simulink model "npc_controller"  (R2022a)
settings: Solver=FixedStepDiscrete  StartTime=0.0  StopTime=20  RelTol=1e-3  EnableMultiTasking=on
undefined symbols (not defined in the file): CAN_O_INT, CANA_BASE, Down, GPTRIP1SEL, GPTRIP2SEL, GPTRIP3SEL, Tsw, TZ1, TZ2, TZ3, Up
libraries: simulink x147, hdlsllib x90, c2802xlib x34, c2837xDlib x20, c280xlib x12, canmsglib x9, c2838xlib x8, idelinklib_common x3, c2806xlib x2, slpidlib x2, c28004xlib x2, c281xlib x2
(part 17 of 42)

== system npc_controller/IDLE_AND_TIMER/codegen/INITIALIZATION/outputxbar ==
  note: Note: GPIO58 is J2.15
  note: //Code:
      | GPIO_setPinConfig(GPIO_24_OUTPUTXBAR1);
      | GPIO_setDirectionMode(24, GPIO_DIR_MODE_OUT);
      | GPIO_setPadConfig(24, GPIO_PIN_TYPE_STD);
      | XBAR_setOutputMuxConfig(XBAR_OUTPUT1, XBAR_OUT_MUX00_CMPSS1_CTRIPOUTH);
      | XBAR_enableOutputMux(XBAR_OUTPUT1, XBAR_MUX00);
      |
      | GPIO_setPinConfig(GPIO_25_OUTPUTXBAR2);
      | GPIO_setDirectionMode(25, GPIO_DIR_MODE_OUT);
      | GPIO_setPadConfig(25, GPIO_PIN_TYPE_STD);
      | XBAR_setOutputMuxConfig(XBAR_OUTPUT2, XBAR_OUT_MUX01_CMPSS1_CTRIPOUTL);
      | XBAR_enableOutputMux(XBAR_OUTPUT2, XBAR_MUX01);
      |
      | GPIO_setPinConfig(GPIO_26_OUTPUTXBAR3);
      | GPIO_setDirectionMode(26, GPIO_DIR_MODE_OUT);
      | GPIO_setPadConfig(26, GPIO_PIN_TYPE_STD);
      | XBAR_setOutputMuxConfig(XBAR_OUTPUT3, XBAR_OUT_MUX04_CMPSS3_CTRIPOUTH);
      | XBAR_enableOutputMux(XBAR_OUTPUT3, XBAR_MUX04);
      |
      | GPIO_setPinConfig(GPIO_27_OUTPUTXBAR4);
      | GPIO_setDirectionMode(27, GPIO_DIR_MODE_OUT);
      | GPIO_setPadConfig(27, GPIO_PIN_TYPE_STD);
      | XBAR_setOutputMuxConfig(XBAR_OUTPUT4, XBAR_OUT_MUX05_CMPSS3_CTRIPOUTL);
      | XBAR_enableOutputMux(XBAR_OUTPUT4, XBAR_MUX05);
  note: GPIO_setPinConfig(GPIO_24_OUTPUTXBAR1);
      | GPIO_setDirectionMode(24, GPIO_DIR_MODE_OUT);
      | GPIO_setPadConfig(24, GPIO_PIN_TYPE_STD);
      | XBAR_setOutputMuxConfig(XBAR_OUTPUT1, XBAR_OUT_MUX11_CMPSS6_CTRIPOUTL);
      | XBAR_enableOutputMux(XBAR_OUTPUT1, XBAR_MUX11);
      |
      | GPIO_setPinConfig(GPIO_25_OUTPUTXBAR2);
      | GPIO_setDirectionMode(25, GPIO_DIR_MODE_OUT);
      | GPIO_setPadConfig(25, GPIO_PIN_TYPE_STD);
      | XBAR_setOutputMuxConfig(XBAR_OUTPUT2, XBAR_OUT_MUX10_CMPSS6_CTRIPOUTH);
      | XBAR_enableOutputMux(XBAR_OUTPUT2, XBAR_MUX10);
  note: GPIO_setPinConfig(GPIO_24_OUTPUTXBAR1);
      | GPIO_setDirectionMode(24, GPIO_DIR_MODE_OUT);
      | GPIO_setPadConfig(24, GPIO_PIN_TYPE_STD);
      | XBAR_setOutputMuxConfig(XBAR_OUTPUT1, XBAR_CLB_MUX08_CMPSS5_CTRIPH);
      | XBAR_enableOutputMux(XBAR_OUTPUT1, XBAR_MUX08);
  note: GPIO_setPinConfig(GPIO_24_OUTPUTXBAR1);
      | GPIO_setDirectionMode(24, GPIO_DIR_MODE_OUT);
      | GPIO_setPadConfig(24, GPIO_PIN_TYPE_STD);
      | XBAR_setOutputMuxConfig(XBAR_OUTPUT1, XBAR_CLB_MUX00_CMPSS1_CTRIPH);
      | XBAR_enableOutputMux(XBAR_OUTPUT1, XBAR_MUX00);
  note: GPIO_setPinConfig(GPIO_25_OUTPUTXBAR2);
      | GPIO_setDirectionMode(25, GPIO_DIR_MODE_OUT);
      | GPIO_setPadConfig(25, GPIO_PIN_TYPE_STD);
      | XBAR_setOutputMuxConfig(XBAR_OUTPUT2, XBAR_CLB_MUX00_CMPSS1_CTRIPH);
      | XBAR_enableOutputMux(XBAR_OUTPUT2, XBAR_MUX00);
  note: GPIO_setPinConfig(GPIO_25_OUTPUTXBAR2);
      | GPIO_setDirectionMode(25, GPIO_DIR_MODE_OUT);
      | GPIO_setPadConfig(25, GPIO_PIN_TYPE_STD);
      | XBAR_setOutputMuxConfig(XBAR_OUTPUT2, XBAR_CLB_MUX08_CMPSS5_CTRIPH);
      | XBAR_enableOutputMux(XBAR_OUTPUT2, XBAR_MUX08);
  note: GPIO_setPinConfig(GPIO_58_OUTPUTXBAR1);
      | GPIO_setDirectionMode(58, GPIO_DIR_MODE_OUT);
      | GPIO_setPadConfig(58, GPIO_PIN_TYPE_STD);
      | XBAR_setOutputMuxConfig(XBAR_OUTPUT1, XBAR_EPWM_MUX00_CMPSS1_CTRIPH);
      | XBAR_enableOutputMux(XBAR_OUTPUT1, XBAR_MUX00);
  function : TriggerPort  TriggerType=function-call  VariantControl=Variant
  System Initialize1 : Subsystem  Commented=on  mask(System Initialize){ShowInLibBrowser=0}
      mask prompts: ShowInLibBrowser "Simulink:masks:CustCodeMaskParam1_MP"
      settings: CopyFcn=cccopyfcn(gcb)  OpenFcn=ccopenfcn('System Initialize Function')
      mask Help: eval('feval(''rtwprivate'',''rtwhelpview'',''rtw_sys_initialize_block'')');
      mask Display: disp('System\nInitialize');
  System Initialize2 : Subsystem  Commented=on  mask(System Initialize){ShowInLibBrowser=0}
      mask prompts: ShowInLibBrowser "Simulink:masks:CustCodeMaskParam1_MP"
      settings: CopyFcn=cccopyfcn(gcb)  OpenFcn=ccopenfcn('System Initialize Function')
      mask Help: eval('feval(''rtwprivate'',''rtwhelpview'',''rtw_sys_initialize_block'')');
      mask Display: disp('System\nInitialize');
  System Initialize3 : Subsystem  Commented=on  mask(System Initialize){ShowInLibBrowser=0}
      mask prompts: ShowInLibBrowser "Simulink:masks:CustCodeMaskParam1_MP"
      settings: CopyFcn=cccopyfcn(gcb)  OpenFcn=ccopenfcn('System Initialize Function')
      mask Help: eval('feval(''rtwprivate'',''rtwhelpview'',''rtw_sys_initialize_block'')');
      mask Display: disp('System\nInitialize');
  System Initialize4 : Subsystem  Commented=on  mask(System Initialize){ShowInLibBrowser=0}
      mask prompts: ShowInLibBrowser "Simulink:masks:CustCodeMaskParam1_MP"
      settings: CopyFcn=cccopyfcn(gcb)  OpenFcn=ccopenfcn('System Initialize Function')
      mask Help: eval('feval(''rtwprivate'',''rtwhelpview'',''rtw_sys_initialize_block'')');
      mask Display: disp('System\nInitialize');
  System Initialize5 : Subsystem  Commented=on  mask(System Initialize){ShowInLibBrowser=0}
      mask prompts: ShowInLibBrowser "Simulink:masks:CustCodeMaskParam1_MP"
      settings: CopyFcn=cccopyfcn(gcb)  OpenFcn=ccopenfcn('System Initialize Function')
      mask Help: eval('feval(''rtwprivate'',''rtwhelpview'',''rtw_sys_initialize_block'')');
      mask Display: disp('System\nInitialize');
  System Initialize6 : Subsystem  Commented=on  mask(System Initialize){ShowInLibBrowser=0}
      mask prompts: ShowInLibBrowser "Simulink:masks:CustCodeMaskParam1_MP"
      settings: CopyFcn=cccopyfcn(gcb)  OpenFcn=ccopenfcn('System Initialize Function')
      mask Help: eval('feval(''rtwprivate'',''rtwhelpview'',''rtw_sys_initialize_block'')');
      mask Display: disp('System\nInitialize');
  System Initialize7 : Subsystem  mask(System Initialize){ShowInLibBrowser=0}
      mask prompts: ShowInLibBrowser "Simulink:masks:CustCodeMaskParam1_MP"
      settings: CopyFcn=cccopyfcn(gcb)  OpenFcn=ccopenfcn('System Initialize Function')
      mask Help: eval('feval(''rtwprivate'',''rtwhelpview'',''rtw_sys_initialize_block'')');
      mask Display: disp('System\nInitialize');

== system npc_controller/IDLE_AND_TIMER/codegen/TIMER_100MS/contstruct_can_msg ==
  note: Format:
      | Byte0 - func_id
      | Byte1 - msb
      | Byte2 - lsb
  func_id : Inport
  data : Inport  Port=2
  Chart : Stateflow chart  TreatAsAtomicUnit=on
  Demux : Demux  Outputs=8
  Display1 : Display  Commented=on
  Display2 : Display  Commented=on
  Scope : Scope  NumInputPorts=3
  can_msg : Outport
  wires:
  func_id/1 -> Display1/1, Chart/1(func_id)
  data/1 -> Display2/1, Chart/2(data)
  Chart/1(can_msg) -> Demux/1, can_msg/1
  Demux/1 -> Scope/1
  Demux/3 -> Scope/3
  Demux/2 -> Scope/2

== system npc_controller/IDLE_AND_TIMER/codegen/TIMER_100MS/get_func_id_data ==
  Cast To Single : DataTypeConversion  Commented=on  OutDataTypeStr=uint16  SaturateOnIntegerOverflow=off  RndMeth=Floor
  Chart2 : Stateflow chart  Commented=on  TreatAsAtomicUnit=on
  Constant : Constant  Value=0  OutDataTypeStr=uint16
  Constant1 : Constant  OutDataTypeStr=uint16
  Constant10 : Constant  Value=6  OutDataTypeStr=uint16
  Constant11 : Constant  Value=7  OutDataTypeStr=uint16
  Constant12 : Constant  Value=8  OutDataTypeStr=uint16
  Constant13 : Constant  Value=9  OutDataTypeStr=uint16
  Constant14 : Constant  Value=0  OutDataTypeStr=uint16
  Constant15 : Constant  Commented=on  Value=69  OutDataTypeStr=uint16
  Constant2 : Constant  Value=2  OutDataTypeStr=uint16
  Constant3 : Constant  Commented=on  Value=2
  Constant4 : Constant  Commented=on  Value=13  OutDataTypeStr=uint16
  Constant5 : Constant  Commented=on  Value=17  OutDataTypeStr=uint16
  Constant6 : Constant  Commented=on  Value=49  OutDataTypeStr=uint16
  Constant7 : Constant  Value=3  OutDataTypeStr=uint16
  Constant8 : Constant  Value=4  OutDataTypeStr=uint16
  Constant9 : Constant  Value=5  OutDataTypeStr=uint16
  Data Store Read : DataStoreRead  DataStoreName=cnt_poll_can_msg  IndexOptions=Index vector (dialog)  Indices=1  OutputSizes=1
  Data Store Read1 : DataStoreRead  DataStoreName=adc_vbulk  IndexOptions=Index vector (dialog)  Indices=1  OutputSizes=1
  Data Store Read10 : DataStoreRead  DataStoreName=adc_ib  IndexOptions=Index vector (dialog)  Indices=1  OutputSizes=1
  Data Store Read11 : DataStoreRead  DataStoreName=adc_ic  IndexOptions=Index vector (dialog)  Indices=1  OutputSizes=1
  Data Store Read12 : DataStoreRead  DataStoreName=status  IndexOptions=Index vector (dialog)  Indices=1  OutputSizes=1
  Data Store Read14 : DataStoreRead  Commented=on  DataStoreName=theta  IndexOptions=Index vector (dialog)  Indices=1  OutputSizes=1
  Data Store Read2 : DataStoreRead  DataStoreName=adc_vmid  IndexOptions=Index vector (dialog)  Indices=1  OutputSizes=1
  Data Store Read3 : DataStoreRead  DataStoreName=adc_va  IndexOptions=Index vector (dialog)  Indices=1  OutputSizes=1
  Data Store Read4 : DataStoreRead  Commented=on  DataStoreName=va  IndexOptions=Index vector (dialog)  Indices=1  OutputSizes=1
  Data Store Read5 : DataStoreRead  Commented=on  DataStoreName=vb  IndexOptions=Index vector (dialog)  Indices=1  OutputSizes=1
  Data Store Read6 : DataStoreRead  Commented=on  DataStoreName=vc  IndexOptions=Index vector (dialog)  Indices=1  OutputSizes=1
  Data Store Read7 : DataStoreRead  DataStoreName=adc_vb  IndexOptions=Index vector (dialog)  Indices=1  OutputSizes=1
  Data Store Read8 : DataStoreRead  DataStoreName=adc_vc  IndexOptions=Index vector (dialog)  Indices=1  OutputSizes=1
  Data Store Read9 : DataStoreRead  DataStoreName=adc_ia  IndexOptions=Index vector (dialog)  Indices=1  OutputSizes=1
  Display : Display
  Multiport Switch : MultiPortSwitch  DataPortOrder=Zero-based contiguous  Inputs=10  DataPortForDefault=Additional data port  DiagnosticForDefault=None  zeroidx=on  SaturateOnIntegerOverflow=off  InputSameDT=off
  Multiport Switch1 : MultiPortSwitch  DataPortOrder=Zero-based contiguous  Inputs=10  DataPortForDefault=Additional data port  DiagnosticForDefault=None  zeroidx=on  SaturateOnIntegerOverflow=off  InputSameDT=off
  Rate Transition : RateTransition  Commented=on
  State Reader : StateReader  Commented=on
  func_id : Outport
  data : Outport  Port=2
  wires:
  Multiport Switch1/1 -> data/1
  Multiport Switch/1 -> Display/1, func_id/1
  Data Store Read/1 -> Multiport Switch/1, Multiport Switch1/1
  Constant/1 -> Multiport Switch/2
  Constant1/1 -> Multiport Switch/3
  Constant2/1 -> Multiport Switch/4
  Constant7/1 -> Multiport Switch/5
  Constant8/1 -> Multiport Switch/6
  Constant9/1 -> Multiport Switch/7
  Constant10/1 -> Multiport Switch/8
  Constant11/1 -> Multiport Switch/9
  Data Store Read3/1 -> Multiport Switch1/2
  Data Store Read7/1 -> Multiport Switch1/3
  Data Store Read8/1 -> Multiport Switch1/4
  Data Store Read9/1 -> Multiport Switch1/5
  Data Store Read10/1 -> Multiport Switch1/6
  Data Store Read1/1 -> Multiport Switch1/8
  Data Store Read11/1 -> Multiport Switch1/7
  Data Store Read2/1 -> Multiport Switch1/9
  Constant12/1 -> Multiport Switch/10
  Data Store Read12/1 -> Multiport Switch1/10
  Constant13/1 -> Multiport Switch/11
  State Reader/1 -> Rate Transition/1
  Cast To Single/1 -> ?
  Rate Transition/1 -> Cast To Single/1
  Constant14/1 -> Multiport Switch1/11

== system npc_controller/IDLE_AND_TIMER/codegen/TIMER_100MS/incr_cnt ==
  Data Store Read : DataStoreRead  DataStoreName=cnt_poll_can_msg  IndexOptions=Index vector (dialog)  Indices=1  OutputSizes=1
  If : If  IfExpression=u1 > 10
  Scope : Scope
  inc : Subsystem  TreatAsAtomicUnit=on
  reset : Subsystem  TreatAsAtomicUnit=on
  wires:
  Data Store Read/1 -> Scope/1, If/1
  If/2 -> inc/Action
  If/1 -> reset/Action

== system npc_controller/IDLE_AND_TIMER/codegen/TIMER_1MS/codegen ==
  periodic_timer1 : Subsystem  TreatAsAtomicUnit=on  ScheduleAs=Periodic partition  PartitionName=timer_1ms  SystemSampleTime=1e-3
      settings: RTWFcnNameOpts=Use subsystem name  RTWFileNameOpts=Use subsystem name

== system npc_controller/IDLE_AND_TIMER/codegen/TIMER_1MS/sim ==

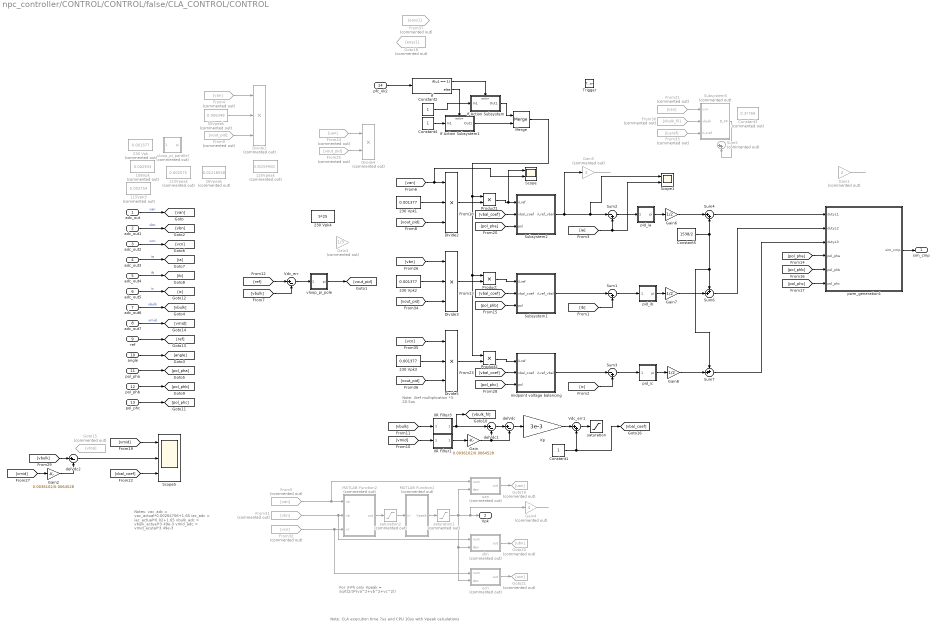
== system npc_controller/CONTROL/CONTROL/false/CLA_CONTROL/CONTROL ==
  note: Note: CLA execution time 7us and CPU 10us with Vpeak calculations
  note: For 3-Ph only
      | Vpeak = sqrt(2/3*(va^2+vb^2+vc^2))
  note: Note:
      | ilref multiplication *3: 20.5us
  note: Notes:
      | vac_adc = vac_actual*0.00264706+1.65
      | iac_adc = iac_actual*0.02+1.65
      | vbulk_adc = vbulk_actual*3.49e-3
      | vmid_adc = vmid_acutal*3.49e-3
  adc_out : Inport  OutDataTypeStr=single
  adc_out1 : Inport  Port=2  OutDataTypeStr=single
  adc_out2 : Inport  Port=3  OutDataTypeStr=single
  adc_out3 : Inport  Port=4  OutDataTypeStr=single
  adc_out4 : Inport  Port=5  OutDataTypeStr=single
  adc_out5 : Inport  Port=6  OutDataTypeStr=single
  adc_out6 : Inport  Port=7  OutDataTypeStr=single
  adc_out7 : Inport  Port=8  OutDataTypeStr=single
  ref : Inport  Port=9
  angle : Inport  Port=10
  pol_pha : Inport  Port=11
  pol_phb : Inport  Port=12
  pol_phc : Inport  Port=13
  pfc_ok2 : Inport  Port=14
  Trigger : TriggerPort  TriggerType=function-call  VariantControl=Variant  PortDimensions=1
  108Vpk : Constant  Commented=on  Value=0.002933  OutDataTypeStr=single
  115Vpk3 : Constant  Commented=on  Value=0.002754  OutDataTypeStr=single
  123Vpeak : Constant  Commented=on  Value=0.002575  OutDataTypeStr=single
  125Vpeak : Constant  Commented=on  Value=0.002534602  OutDataTypeStr=single
  230 Vpk : Constant  Commented=on  Value=0.001377  OutDataTypeStr=single
  230 Vpk1 : Constant  Value=0.001377  OutDataTypeStr=single
  230 Vpk2 : Constant  Value=0.001377  OutDataTypeStr=single
  230 Vpk3 : Constant  Value=0.001377  OutDataTypeStr=single
  230 Vpk4 : Constant  Value=5*25  OutDataTypeStr=single
  26Vpeak : Constant  Commented=on  Value=0.01218558  OutDataTypeStr=single
  50Vpeak : Constant  Commented=on  Value=0.006348  OutDataTypeStr=single
  Constant1 : Constant  OutDataTypeStr=single  SampleTime=-1
  Constant2 : Constant  OutDataTypeStr=single
  Constant3 : Constant  Commented=on  Value=0.3*769  OutDataTypeStr=single  SampleTime=-1
  Constant4 : Constant  OutDataTypeStr=single
  Constant5 : Constant  Value=1538/2  OutDataTypeStr=single  SampleTime=-1
  Divide1 : Product  Commented=on  Inputs=***  OutDataTypeStr=single
  Divide2 : Product  Inputs=***  OutDataTypeStr=single
  Divide3 : Product  Inputs=***  OutDataTypeStr=single
  Divide4 : Product  Commented=on  Inputs=**  OutDataTypeStr=single
  Divide5 : Product  Inputs=***  OutDataTypeStr=single
  From21 : From  Commented=on  GotoTag=van
  From24 : From  Commented=on  GotoTag=uan
  From25 : From  Commented=on  GotoTag=vout_pid
  From30 : From  Commented=on  GotoTag=vbulk_fil
  From31 : From  Commented=on  GotoTag=vbn
  From32 : From  Commented=on  GotoTag=vcn
  From33 : From  Commented=on  GotoTag=iLaref
  From37 : From  Commented=on  GotoTag=eoss1
  From4 : From  Commented=on  GotoTag=van
  From5 : From  Commented=on  GotoTag=van
  From9 : From  Commented=on  GotoTag=vout_pid
  Gain : Gain  Gain=0.0036102/0.0064528
  Gain1 : Gain  Commented=on  Gain=2  ParamDataTypeStr=single  OutDataTypeStr=single
  Gain2 : Gain  Gain=0.0036102/0.0064528
  Gain3 : Gain  Commented=on  Gain=1/3  ParamDataTypeStr=single  OutDataTypeStr=single
  Gain4 : Gain  Commented=on  Gain=4  ParamDataTypeStr=single  OutDataTypeStr=single
  Gain5 : Gain  Commented=on  Gain=3  ParamDataTypeStr=single  OutDataTypeStr=single
  Gain6 : Gain  Gain=1/2  ParamDataTypeStr=single  OutDataTypeStr=single
  Gain7 : Gain  Gain=1/2  ParamDataTypeStr=single  OutDataTypeStr=single
  Gain8 : Gain  Gain=1/2  ParamDataTypeStr=single  OutDataTypeStr=single
  Goto15 : Goto  Commented=on  GotoTag=vtop
  Goto18 : Goto  Commented=on  GotoTag=eoss1
  Goto19 : Goto  Commented=on  GotoTag=uan
  Goto20 : Goto  Commented=on  GotoTag=ubn
  Goto21 : Goto  Commented=on  GotoTag=ucn
  IIR Filter1 : Subsystem
  IIR Filter3 : Subsystem
  If : If  IfExpression=u1 == 1
  If Action Subsystem : Subsystem  TreatAsAtomicUnit=on
  If Action Subsystem1 : Subsystem  TreatAsAtomicUnit=on
  Kp : Gain  Gain=3e-3  ParamDataTypeStr=single  OutDataTypeStr=single
  MATLAB Function1 : MATLAB Function  Commented=on  TreatAsAtomicUnit=on
  MATLAB Function2 : MATLAB Function  Commented=on  TreatAsAtomicUnit=on
  Merge : Merge  InitialOutput=[0.25]
  Product : Product  OutDataTypeStr=single
  Product1 : Product  OutDataTypeStr=single
  Product2 : Product  OutDataTypeStr=single
  Scope : Scope  NumInputPorts=2
  Scope1 : Scope  NumInputPorts=2
  Scope5 : Scope  NumInputPorts=3
  Subsystem1 : Subsystem
  Subsystem2 : Subsystem
  Subsystem5 : Subsystem  Commented=on
  Sum1 : Sum  Inputs=|-+  AccumDataTypeStr=single  OutDataTypeStr=single
  Sum2 : Sum  Inputs=|-+  AccumDataTypeStr=single  OutDataTypeStr=single
  Sum3 : Sum  Inputs=|-+  AccumDataTypeStr=single  OutDataTypeStr=single
  Sum4 : Sum  Inputs=|++  AccumDataTypeStr=single  OutDataTypeStr=single
  Sum5 : Sum  Commented=on  Inputs=|++  AccumDataTypeStr=single  OutDataTypeStr=single
  Sum6 : Sum  Inputs=++|  AccumDataTypeStr=single  OutDataTypeStr=single
  Sum7 : Sum  Inputs=++|  AccumDataTypeStr=single  OutDataTypeStr=single
  Vdc_err : Sum  Inputs=|+-  AccumDataTypeStr=single  OutDataTypeStr=single
  Vdc_err1 : Sum  Inputs=|++  AccumDataTypeStr=single  OutDataTypeStr=single
  delVdc : Sum  Inputs=|+-  AccumDataTypeStr=single  OutDataTypeStr=single
  delVdc1 : Sum  Inputs=|+-  AccumDataTypeStr=single  OutDataTypeStr=single
  delVdc2 : Sum  Inputs=|+-  AccumDataTypeStr=single  OutDataTypeStr=single
  midpoint voltage balancing : Subsystem
  pid_ia : Subsystem
      mask Display: disp('PID(z)')
  pid_ib : Subsystem
      mask Display: disp('PID(z)')
  pid_ic : Subsystem
      mask Display: disp('PID(z)')
  pwm_generation1 : Subsystem
  saturation : Saturate  UpperLimit=1.8  LowerLimit=0.2  OutDataTypeStr=single
  saturation1 : Saturate  Commented=on  UpperLimit=inf  LowerLimit=1  OutDataTypeStr=single
  saturation2 : Saturate  Commented=on  UpperLimit=inf  LowerLimit=1  OutDataTypeStr=single
  uan : MATLAB Function  Priority=2  Commented=on  TreatAsAtomicUnit=on
      settings: RTWSystemCode=Inline
  ubn : MATLAB Function  Priority=2  Commented=on  TreatAsAtomicUnit=on
      settings: RTWSystemCode=Inline
  ucn : MATLAB Function  Priority=2  Commented=on  TreatAsAtomicUnit=on
      settings: RTWSystemCode=Inline
  vloop_pi_parallel : Subsystem  Commented=on
      mask Display: disp('PID(z)')
  vloop_pi_pole : Subsystem
      mask Display: disp('PID(z)')
  sim_cmp : Outport
  Vpk : Outport  Port=2
  wires:
  adc_out3/1 -> [ia]  "ia"
  adc_out2/1 -> [vcn]  "vcn"
  adc_out/1 -> [van]  "van"
  adc_out5/1 -> [ic]  "ic"
  adc_out1/1 -> [vbn]  "vbn"
  adc_out4/1 -> [ib]  "ib"
  adc_out6/1 -> [vbulk]  "vbulk"
  adc_out7/1 -> [vmid]  "vmid"
  [ic] -> Sum3/2
  Vdc_err/1 -> vloop_pi_pole/1(error)
  [ib] -> Sum1/2
  From4/1 -> Divide1/1
  50Vpeak/1 -> Divide1/2
  Kp/1 -> Vdc_err1/1
  delVdc1/1 -> delVdc/1
  delVdc/1 -> Kp/1
  midpoint voltage balancing/1(iLref_vbal) -> Sum3/1
  pwm_generation1/1(sim_cmp) -> sim_cmp/1
  ref/1 -> [ref]
  Sum2/1 -> pid_ia/1(error)
  Sum1/1 -> pid_ib/1(error)
  Sum3/1 -> pid_ic/1(error)
  Subsystem2/1(iLref_vbal) -> Gain5/1, Scope1/1, Sum2/1
  [ia] -> Scope1/2, Sum2/2
  pid_ic/1(pi) -> Gain8/1
  [pol_phc] -> pwm_generation1/6(pol_phc)
  [pol_phb] -> pwm_generation1/5(pol_phb)
  [pol_pha] -> pwm_generation1/4(pol_pha)
  pol_pha/1 -> [pol_pha]
  pol_phb/1 -> [pol_phb]
  pol_phc/1 -> [pol_phc]
  Vdc_err1/1 -> saturation/1
  Constant1/1 -> [vbal_coef], Vdc_err1/2
  [vbal_coef] -> Scope5/3
  [pol_phc] -> midpoint voltage balancing/3(pol)
  [vbal_coef] -> midpoint voltage balancing/2(vbal_coef)
  [vbal_coef] -> Subsystem1/2(vbal_coef)
  [pol_phb] -> Subsystem1/3(pol)
  [pol_pha] -> Subsystem2/3(pol)
  [vbal_coef] -> Subsystem2/2(vbal_coef)
  angle/1 -> [angle]
  From25/1 -> Divide4/2
  pid_ib/1(pi) -> Gain7/1
  Subsystem1/1(iLref_vbal) -> Sum1/1
  delVdc2/1 -> Scope5/2
  [vmid] -> Scope5/1
  [vmid] -> Gain2/1
  [vbulk] -> delVdc2/1
  [vmid] -> IIR Filter1/1(x[n])
  Gain/1 -> delVdc1/2, delVdc/2
  Gain2/1 -> delVdc2/2
  [vbulk] -> IIR Filter3/1(x[n])
  From21/1 -> Subsystem5/1(vxn)
  From30/1 -> Subsystem5/2(vbulk)
  From33/1 -> Subsystem5/3(iLxref)
  Subsystem5/1(D_FF) -> Sum5/2
  IIR Filter1/1(y[n]) -> Gain/1
  IIR Filter3/1(y[n]) -> [vbulk_fil], delVdc1/1
  pid_ia/1(pi) -> Gain6/1
  [vbulk] -> Vdc_err/2
  Gain1/1 -> ?
  uan/1(out) -> Goto19/1
  ucn/1(out) -> Goto21/1
  From31/1 -> ubn/1(num), MATLAB Function2/2(vb)
  From5/1 -> uan/1(num), MATLAB Function2/1(va)
  From32/1 -> ucn/1(num), MATLAB Function2/3(vc)
  MATLAB Function1/1(Vpeak) -> saturation1/1
  MATLAB Function2/1(out) -> saturation2/1
  ubn/1(out) -> Goto20/1
  From24/1 -> Divide4/1
  Gain4/1 -> ?
  Gain5/1 -> ?
  Divide3/1 -> Product/2
  Product/1 -> Subsystem1/1(iLref)
  If/1 -> If Action Subsystem/Action
  Constant2/1 -> If Action Subsystem/1(In1)
  If/2 -> If Action Subsystem1/Action
  Constant4/1 -> If Action Subsystem1/1(In1)
  If Action Subsystem/1(Out1) -> Merge/1
  If Action Subsystem1/1(Out1) -> Merge/2
  Merge/1 -> Product1/1, Product2/1, Product/1
  pfc_ok2/1 -> If/1
  Divide2/1 -> Product1/2
  Product1/1 -> Scope/1, Subsystem2/1(iLref)
  Divide5/1 -> Product2/2
  Product2/1 -> midpoint voltage balancing/1(iLref)
  [ref] -> Vdc_err/1
  From9/1 -> Divide1/3
  saturation1/1 -> Gain4/1, Vpk/1, ucn/2(den), ubn/2(den), uan/2(den)
  saturation2/1 -> MATLAB Function1/1(in)
  [vout_pid] -> Divide2/3
  230 Vpk1/1 -> Divide2/2
  [van] -> Scope/2, Divide2/1
  [vbn] -> Divide3/1
  230 Vpk2/1 -> Divide3/2
  [vout_pid] -> Divide3/3
  [vout_pid] -> Divide5/3
  230 Vpk3/1 -> Divide5/2
  [vcn] -> Divide5/1
  Gain6/1 -> Sum4/1
  Constant5/1 -> Sum7/1, Sum6/1, Sum4/2
  Gain7/1 -> Sum6/2
  Gain8/1 -> Sum7/2
  Sum6/1 -> pwm_generation1/2(dutyL2)
  Sum7/1 -> pwm_generation1/3(dutyL3)
  vloop_pi_pole/1(pi) -> [vout_pid]
  Sum4/1 -> pwm_generation1/1(dutyL1)

== system npc_controller/CONTROL/CONTROL/false/CLA_CONTROL/GPIO_HIGH ==
  Trigger : TriggerPort  TriggerType=function-call  VariantControl=Variant  PortDimensions=1
  Constant1 : Constant  Commented=on  OutDataTypeStr=single
  Constant2 : Constant  Commented=on  OutDataTypeStr=single
  GPIO139_J5.43 : c2838xlib/Digital Output  Commented=on  GPIO_Number=GPIO136~GPIO143  GPIO_Bit0=off  GPIO_BIT0_Toggle=off  GPIO_Bit1=off  GPIO_BIT1_Toggle=off  GPIO_Bit2=off  GPIO_BIT2_Toggle=off  GPIO_Bit3=on  GPIO_BIT3_Toggle=off  GPIO_Bit4=off  GPIO_BIT4_Toggle=off  GPIO_Bit5=off  GPIO_BIT5_Toggle=off  GPIO_Bit6=off  GPIO_BIT6_Toggle=off  GPIO_Bit7=off  GPIO_BIT7_Toggle=off
      settings: SourceProductBaseCode=TIC2000
  GPIO58.PFC_OK : c2838xlib/Digital Output  Commented=on  GPIO_Number=GPIO56~GPIO63  GPIO_Bit0=off  GPIO_BIT0_Toggle=off  GPIO_Bit1=off  GPIO_BIT1_Toggle=off  GPIO_Bit2=on  GPIO_BIT2_Toggle=off  GPIO_Bit3=off  GPIO_BIT3_Toggle=off  GPIO_Bit4=off  GPIO_BIT4_Toggle=off  GPIO_Bit5=off  GPIO_BIT5_Toggle=off  GPIO_Bit6=off  GPIO_BIT6_Toggle=off  GPIO_Bit7=off  GPIO_BIT7_Toggle=off
      settings: SourceProductBaseCode=TIC2000
  wires:
  Constant1/1 -> GPIO139_J5.43/1
  Constant2/1 -> GPIO58.PFC_OK/1

== system npc_controller/CONTROL/CONTROL/false/CLA_CONTROL/GPIO_LOW ==
  Trigger : TriggerPort  TriggerType=function-call  VariantControl=Variant  PortDimensions=1
  Constant1 : Constant  Commented=on  Value=0  OutDataTypeStr=single
  Constant3 : Constant  Commented=on  Value=0  OutDataTypeStr=single
  GPIO139_J5.43 : c2838xlib/Digital Output  Commented=on  GPIO_Number=GPIO136~GPIO143  GPIO_Bit0=off  GPIO_BIT0_Toggle=off  GPIO_Bit1=off  GPIO_BIT1_Toggle=off  GPIO_Bit2=off  GPIO_BIT2_Toggle=off  GPIO_Bit3=on  GPIO_BIT3_Toggle=off  GPIO_Bit4=off  GPIO_BIT4_Toggle=off  GPIO_Bit5=off  GPIO_BIT5_Toggle=off  GPIO_Bit6=off  GPIO_BIT6_Toggle=off  GPIO_Bit7=off  GPIO_BIT7_Toggle=off
      settings: SourceProductBaseCode=TIC2000
  GPIO58.PFC_OK : c2838xlib/Digital Output  Commented=on  GPIO_Number=GPIO56~GPIO63  GPIO_Bit0=off  GPIO_BIT0_Toggle=off  GPIO_Bit1=off  GPIO_BIT1_Toggle=off  GPIO_Bit2=on  GPIO_BIT2_Toggle=off  GPIO_Bit3=off  GPIO_BIT3_Toggle=off  GPIO_Bit4=off  GPIO_BIT4_Toggle=off  GPIO_Bit5=off  GPIO_BIT5_Toggle=off  GPIO_Bit6=off  GPIO_BIT6_Toggle=off  GPIO_Bit7=off  GPIO_BIT7_Toggle=off
      settings: SourceProductBaseCode=TIC2000
  wires:
  Constant3/1 -> GPIO139_J5.43/1
  Constant1/1 -> GPIO58.PFC_OK/1

== system npc_controller/CONTROL/CONTROL/false/CLA_CONTROL/INIT//RESET_CONTROL ==
  control_en : Inport
  pha_en1 : Inport  Port=2
  phb_en1 : Inport  Port=3
  phc_en1 : Inport  Port=4
  Trigger : TriggerPort  TriggerType=function-call  VariantControl=Variant  PortDimensions=1
  If : If  NumInputs=3  IfExpression=(u1 & u2 & u3) == 1
  If1 : If  IfExpression=u1 == 0
  If2 : If  IfExpression=u1 == 0
  If3 : If  IfExpression=u1 == 0
  NOT : Logic  Operator=NOT  IconShape=distinctive  AllPortsSameDT=off  OutDataTypeStr=boolean
  NOT1 : Logic  Operator=NOT  IconShape=distinctive  AllPortsSameDT=off  OutDataTypeStr=boolean
  NOT2 : Logic  Operator=NOT  IconShape=distinctive  AllPortsSameDT=off  OutDataTypeStr=boolean
  true : Subsystem  TreatAsAtomicUnit=on
      settings: RTWSystemCode=Inline
  true1 : Subsystem  TreatAsAtomicUnit=on
      settings: RTWSystemCode=Inline
  true2 : Subsystem  TreatAsAtomicUnit=on
      settings: RTWSystemCode=Inline
  true3 : Subsystem  TreatAsAtomicUnit=on
      settings: RTWSystemCode=Inline
  wires:
  NOT/1 -> If/1
  NOT1/1 -> If/2
  If1/1 -> true1/Action
  NOT2/1 -> If/3
  phb_en1/1 -> NOT1/1, If2/1
  phc_en1/1 -> NOT2/1, If3/1
  If2/1 -> true2/Action
  If3/1 -> true3/Action
  pha_en1/1 -> NOT/1, If1/1
  If/1 -> true/Action

== system npc_controller/CONTROL/GET_ADC/ADC/codegen/ADCA ==
  note: Note:
      | A0 VCSB_AD J3.30
      | A1 T_MUX_AD J7.70
      | A2 ICSC_AD J3.29
      | A3 VSCC_AD J3.26
      | A4 ICSA_AD J7.69
      | A5 VCSA_AD J7.66
      |
      | 14 ICSB_AD J3.23
      | 15 VBIAS_AD J7.63
      |
      | B0 IPHASE_A_ADC XX
      | B1 ADC_DEBUG_1 XX
      | B2 IPHASE_B_ADC J3.28
      | B3 IPHASE_C_ADC J3.25
      | B4 VPFC_OUT_AD J7.68
      | B5 VPFC_MID_AD J7.65
      |
      | *Near grid is ics
  Trigger : TriggerPort  TriggerType=function-call  VariantControl=(inherit)  PortDimensions=1
  ADC17 : c2802xlib/ADC  blkParamProc=C2000_Type4  ADCModule=A  samplingMode=Single sample mode  ADCResolution=12-bit (Single-ended input)  useSOC1=SOC6  useSOC2=SOC0_SOC1  SOCAcquisitionWindow=15  SOCTriggerSource=ePWM1_ADCSOCA  SOCInterruptTrigger=No ADCINT  Ts=-1  dType=single  postInterrupt=off  interruptSel=ADCINT1  ADCINTContinuous=off  endma=off  chdma=1  conv1=ADCINA0  conv2=ADCINA0 and ADCINB0  conv1_Type4=ADCIN14  conv2_Type4=ADCIN0 and ADCIN1
  ADC18 : c2802xlib/ADC  blkParamProc=C2000_Type4  ADCModule=A  samplingMode=Single sample mode  ADCResolution=12-bit (Single-ended input)  useSOC1=SOC0  useSOC2=SOC0_SOC1  SOCAcquisitionWindow=15  SOCTriggerSource=ePWM1_ADCSOCA  SOCInterruptTrigger=No ADCINT  Ts=-1  dType=single  postInterrupt=off  interruptSel=ADCINT1  ADCINTContinuous=off  endma=off  chdma=1  conv1=ADCINA0  conv2=ADCINA0 and ADCINB0  conv1_Type4=ADCIN0  conv2_Type4=ADCIN0 and ADCIN1
  ADC3 : c2802xlib/ADC  blkParamProc=C2000_Type4  ADCModule=A  samplingMode=Single sample mode  ADCResolution=12-bit (Single-ended input)  useSOC1=SOC2  useSOC2=SOC0_SOC1  SOCAcquisitionWindow=15  SOCTriggerSource=ePWM1_ADCSOCA  SOCInterruptTrigger=No ADCINT  Ts=-1  dType=single  postInterrupt=off  interruptSel=ADCINT1  ADCINTContinuous=off  endma=off  chdma=1  conv1=ADCINA0  conv2=ADCINA0 and ADCINB0  conv1_Type4=ADCIN2  conv2_Type4=ADCIN0 and ADCIN1
  ADC4 : c2802xlib/ADC  Commented=on  blkParamProc=C2000_Type4  ADCModule=A  samplingMode=Single sample mode  ADCResolution=12-bit (Single-ended input)  useSOC1=SOC1  useSOC2=SOC0_SOC1  SOCAcquisitionWindow=15  SOCTriggerSource=ePWM1_ADCSOCA  SOCInterruptTrigger=No ADCINT  Ts=-1  dType=single  postInterrupt=off  interruptSel=ADCINT1  ADCINTContinuous=off  endma=off  chdma=1  conv1=ADCINA0  conv2=ADCINA0 and ADCINB0  conv1_Type4=ADCIN1  conv2_Type4=ADCIN0 and ADCIN1
  ADC5 : c2802xlib/ADC  blkParamProc=C2000_Type4  ADCModule=A  samplingMode=Single sample mode  ADCResolution=12-bit (Single-ended input)  useSOC1=SOC4  useSOC2=SOC0_SOC1  SOCAcquisitionWindow=15  SOCTriggerSource=ePWM1_ADCSOCA  SOCInterruptTrigger=No ADCINT  Ts=-1  dType=single  postInterrupt=off  interruptSel=ADCINT1  ADCINTContinuous=off  endma=off  chdma=1  conv1=ADCINA0  conv2=ADCINA0 and ADCINB0  conv1_Type4=ADCIN4  conv2_Type4=ADCIN0 and ADCIN1
  ADC6 : c2802xlib/ADC  blkParamProc=C2000_Type4  ADCModule=A  samplingMode=Single sample mode  ADCResolution=12-bit (Single-ended input)  useSOC1=SOC5  useSOC2=SOC0_SOC1  SOCAcquisitionWindow=15  SOCTriggerSource=ePWM1_ADCSOCA  SOCInterruptTrigger=No ADCINT  Ts=-1  dType=single  postInterrupt=off  interruptSel=ADCINT1  ADCINTContinuous=off  endma=off  chdma=1  conv1=ADCINA0  conv2=ADCINA0 and ADCINB0  conv1_Type4=ADCIN5  conv2_Type4=ADCIN0 and ADCIN1
  ADC7 : c2802xlib/ADC  blkParamProc=C2000_Type4  ADCModule=A  samplingMode=Single sample mode  ADCResolution=12-bit (Single-ended input)  useSOC1=SOC3  useSOC2=SOC0_SOC1  SOCAcquisitionWindow=15  SOCTriggerSource=ePWM1_ADCSOCA  SOCInterruptTrigger=No ADCINT  Ts=-1  dType=single  postInterrupt=off  interruptSel=ADCINT1  ADCINTContinuous=off  endma=off  chdma=1  conv1=ADCINA0  conv2=ADCINA0 and ADCINB0  conv1_Type4=ADCIN3  conv2_Type4=ADCIN0 and ADCIN1
  ADC8 : c2802xlib/ADC  blkParamProc=C2000_Type4  ADCModule=A  samplingMode=Single sample mode  ADCResolution=12-bit (Single-ended input)  useSOC1=SOC7  useSOC2=SOC0_SOC1  SOCAcquisitionWindow=15  SOCTriggerSource=ePWM1_ADCSOCA  SOCInterruptTrigger=No ADCINT  Ts=-1  dType=single  postInterrupt=on  interruptSel=ADCINT1  ADCINTContinuous=on  endma=off  chdma=1  conv1=ADCINA0  conv2=ADCINA0 and ADCINB0  conv1_Type4=ADCIN15  conv2_Type4=ADCIN0 and ADCIN1
  Subsystem10 : Subsystem
  Subsystem11 : Subsystem
  Subsystem17 : Subsystem  Commented=on
  Subsystem18 : Subsystem
  Subsystem6 : Subsystem
  Subsystem7 : Subsystem
  Subsystem8 : Subsystem
  Subsystem9 : Subsystem
  vb : Outport
  ic : Outport  Port=2
  vc : Outport  Port=3
  ia : Outport  Port=4
  va : Outport  Port=5
  ib : Outport  Port=6
  wires:
  ADC7/1 -> Subsystem11/1(x[n])
  ADC18/1 -> Subsystem10/1(In1)
  ADC8/1 -> Subsystem18/1(In1)
  ADC17/1 -> Subsystem7/1(x[n])
  Subsystem8/1(Outport) -> ia/1
  ADC4/1 -> Subsystem17/1(Inport)
  ADC6/1 -> Subsystem9/1(x[n])
  Subsystem6/1(Outport) -> ic/1
  Subsystem11/1(Outport) -> vc/1
  Subsystem7/1(Outport) -> ib/1
  Subsystem10/1(Outport) -> vb/1
  Subsystem9/1(Outport) -> va/1
  ADC5/1 -> Subsystem6/1(Input)
  ADC3/1 -> Subsystem8/1(Input)

== system npc_controller/CONTROL/GET_ADC/ADC/codegen/ADCC ==
  note: for dacc
  Trigger : TriggerPort  TriggerType=function-call  VariantControl=(inherit)  PortDimensions=1
  ADC1 : c2802xlib/ADC  Commented=on  blkParamProc=C2000_Type4  ADCModule=B  samplingMode=Single sample mode  ADCResolution=12-bit (Single-ended input)  useSOC1=SOC1  useSOC2=SOC0_SOC1  SOCAcquisitionWindow=15  SOCTriggerSource=Software  SOCInterruptTrigger=No ADCINT  Ts=-1  dType=single  postInterrupt=off  interruptSel=ADCINT1  ADCINTContinuous=off  endma=off  chdma=1  conv1=ADCINA0  conv2=ADCINA0 and ADCINB0  conv1_Type4=ADCIN1  conv2_Type4=ADCIN0 and ADCIN1
  ADC2 : c2802xlib/ADC  blkParamProc=C2000_Type4  ADCModule=B  samplingMode=Single sample mode  ADCResolution=12-bit (Single-ended input)  useSOC1=SOC1  useSOC2=SOC0_SOC1  SOCAcquisitionWindow=15  SOCTriggerSource=Software  SOCInterruptTrigger=No ADCINT  Ts=-1  dType=single  postInterrupt=off  interruptSel=ADCINT1  ADCINTContinuous=off  endma=off  chdma=1  conv1=ADCINA0  conv2=ADCINA0 and ADCINB0  conv1_Type4=ADCIN2  conv2_Type4=ADCIN0 and ADCIN1
  ADC3 : c2802xlib/ADC  blkParamProc=C2000_Type4  ADCModule=B  samplingMode=Single sample mode  ADCResolution=12-bit (Single-ended input)  useSOC1=SOC3  useSOC2=SOC0_SOC1  SOCAcquisitionWindow=15  SOCTriggerSource=Software  SOCInterruptTrigger=No ADCINT  Ts=-1  dType=single  postInterrupt=off  interruptSel=ADCINT1  ADCINTContinuous=off  endma=off  chdma=1  conv1=ADCINA0  conv2=ADCINA0 and ADCINB0  conv1_Type4=ADCIN4  conv2_Type4=ADCIN0 and ADCIN1
  ADC4 : c2802xlib/ADC  blkParamProc=C2000_Type4  ADCModule=B  samplingMode=Single sample mode  ADCResolution=12-bit (Single-ended input)  useSOC1=SOC4  useSOC2=SOC0_SOC1  SOCAcquisitionWindow=15  SOCTriggerSource=Software  SOCInterruptTrigger=No ADCINT  Ts=-1  dType=single  postInterrupt=off  interruptSel=ADCINT1  ADCINTContinuous=off  endma=off  chdma=1  conv1=ADCINA0  conv2=ADCINA0 and ADCINB0  conv1_Type4=ADCIN5  conv2_Type4=ADCIN0 and ADCIN1
  ADC5 : c2802xlib/ADC  blkParamProc=C2000_Type4  ADCModule=B  samplingMode=Single sample mode  ADCResolution=12-bit (Single-ended input)  useSOC1=SOC2  useSOC2=SOC0_SOC1  SOCAcquisitionWindow=15  SOCTriggerSource=Software  SOCInterruptTrigger=No ADCINT  Ts=-1  dType=single  postInterrupt=off  interruptSel=ADCINT1  ADCINTContinuous=off  endma=off  chdma=1  conv1=ADCINA0  conv2=ADCINA0 and ADCINB0  conv1_Type4=ADCIN3  conv2_Type4=ADCIN0 and ADCIN1
  ADC6 : c2802xlib/ADC  blkParamProc=C2000_Type4  ADCModule=B  samplingMode=Single sample mode  ADCResolution=12-bit (Single-ended input)  useSOC1=SOC0  useSOC2=SOC0_SOC1  SOCAcquisitionWindow=15  SOCTriggerSource=Software  SOCInterruptTrigger=No ADCINT  Ts=-1  dType=single  postInterrupt=off  interruptSel=ADCINT1  ADCINTContinuous=off  endma=off  chdma=1  conv1=ADCINA0  conv2=ADCINA0 and ADCINB0  conv1_Type4=ADCIN0  conv2_Type4=ADCIN0 and ADCIN1
  Subsystem12 : Subsystem
  Subsystem13 : Subsystem
  Subsystem14 : Subsystem
  Subsystem15 : Subsystem
  Subsystem16 : Subsystem
  iphasea : Outport
  iphaseb : Outport  Port=2
  iphasec : Outport  Port=3
  vbulk : Outport  Port=4
  vmid : Outport  Port=5
  wires:
  ADC2/1 -> Subsystem15/1(In1)
  Subsystem13/1(Outport) -> vbulk/1
  ADC3/1 -> Subsystem13/1(x[n])
  Subsystem12/1(Outport) -> vmid/1
  ADC4/1 -> Subsystem12/1(In1)
  ADC5/1 -> Subsystem16/1(In1)
  ADC6/1 -> Subsystem14/1(In1)
  Subsystem14/1(iphasea) -> iphasea/1
  Subsystem16/1(iphasec) -> iphasec/1
  Subsystem15/1(iphaseb) -> iphaseb/1

== system npc_controller/CONTROL/GET_ADC/ADC/codegen/IIR Filter7 ==
  note: prev 0.98
  x[n] : Inport
  1 - Lambda : Gain  Gain=1 - 0.95  ParamDataTypeStr=single  OutDataTypeStr=single
  Delay : Delay  DelayLength=1
  Lambda : Gain  Gain=0.95  ParamDataTypeStr=single  OutDataTypeStr=single
  Sum : Sum  Inputs=|++  AccumDataTypeStr=single  OutDataTypeStr=single
  y[n] : Outport
  wires:
  Delay/1 -> Lambda/1
  Lambda/1 -> Sum/2
  Sum/1 -> y[n]/1, Delay/1
  1 - Lambda/1 -> Sum/1
  x[n]/1 -> 1 - Lambda/1

== system npc_controller/CONTROL/GET_ADC/ADC/codegen/If Action Subsystem ==
  Action Port : ActionPort  ActionPortLabel=if(u1 < 100 & u2 < 100 & u3 < 100)
  Constant : Constant  Value=0  OutDataTypeStr=boolean
  Out1 : Outport
  wires:
  Constant/1 -> Out1/1

== system npc_controller/CONTROL/GET_ADC/ADC/codegen/If Action Subsystem1 ==
  Action Port : ActionPort  ActionPortLabel=if(u1 > 134 & u2 > 134 & u3 > 134)
  Constant : Constant  Value=0  OutDataTypeStr=boolean
  Out1 : Outport
  wires:
  Constant/1 -> Out1/1

== system npc_controller/CONTROL/GET_ADC/ADC/codegen/If Action Subsystem2 ==
  Action Port : ActionPort  ActionPortLabel=else
  Constant : Constant  OutDataTypeStr=boolean
  Out1 : Outport
  wires:
  Constant/1 -> Out1/1

== system npc_controller/CONTROL/GET_ADC/ADC/codegen/If Action Subsystem3 ==
  Action Port : ActionPort  ActionPortLabel=else
  Constant : Constant  OutDataTypeStr=boolean
  Out1 : Outport
  wires:
  Constant/1 -> Out1/1

== system npc_controller/CONTROL/GET_ADC/ADC/codegen/Subsystem ==
  note: ave to rms
  adc : Inport
  Data Store Write3 : DataStoreWrite  DataStoreName=rms_va  IndexOptions=Index vector (dialog)  Indices=1  OutputSizes=1
  Gain : Gain  Gain=1.11  ParamDataTypeStr=single  OutDataTypeStr=single
  IIR Filter1 : Subsystem
  Less Than : RelationalOperator  Operator=>  OutDataTypeStr=boolean  RndMeth=Simplest  InputSameDT=off
  Less Than1 : RelationalOperator  Operator=<  OutDataTypeStr=boolean  RndMeth=Simplest  InputSameDT=off
  Offset7 : Constant  Value=0  OutDataTypeStr=single
  Offset8 : Constant  Value=0  OutDataTypeStr=single
  Product : Product  OutDataTypeStr=single
  Product1 : Product  OutDataTypeStr=single
  vabc7 : Sum  Inputs=|+-  AccumDataTypeStr=single  OutDataTypeStr=single
  adc_rect : Outport
  wires:
  Less Than1/1 -> Product1/2
  Offset7/1 -> Less Than/2
  Offset8/1 -> Less Than1/2
  Less Than/1 -> Product/2
  Product/1 -> vabc7/1
  Product1/1 -> vabc7/2
  adc/1 -> Product1/1, Less Than1/1, Product/1, Less Than/1
  vabc7/1 -> IIR Filter1/1(x[n]), adc_rect/1
  IIR Filter1/1(y[n]) -> Gain/1  "va"
  Gain/1 -> Data Store Write3/1

== system npc_controller/CONTROL/GET_ADC/ADC/codegen/Subsystem1 ==
  adc : Inport
  Data Store Write3 : DataStoreWrite  DataStoreName=rms_vb  IndexOptions=Index vector (dialog)  Indices=1  OutputSizes=1
  Gain : Gain  Gain=1.11  ParamDataTypeStr=single  OutDataTypeStr=single
  IIR Filter1 : Subsystem
  Less Than : RelationalOperator  Operator=>  OutDataTypeStr=boolean  RndMeth=Simplest  InputSameDT=off
  Less Than1 : RelationalOperator  Operator=<  OutDataTypeStr=boolean  RndMeth=Simplest  InputSameDT=off
  Offset7 : Constant  Value=0  OutDataTypeStr=single
  Offset8 : Constant  Value=0  OutDataTypeStr=single
  Product : Product  OutDataTypeStr=single
  Product1 : Product  OutDataTypeStr=single
  vabc7 : Sum  Inputs=|+-  AccumDataTypeStr=single  OutDataTypeStr=single
  adc_rect : Outport
  wires:
  vabc7/1 -> IIR Filter1/1(x[n]), adc_rect/1
  adc/1 -> Less Than/1, Product/1, Less Than1/1, Product1/1
  Product1/1 -> vabc7/2
  Product/1 -> vabc7/1
  Less Than/1 -> Product/2
  Offset8/1 -> Less Than1/2
  Offset7/1 -> Less Than/2
  Less Than1/1 -> Product1/2
  IIR Filter1/1(y[n]) -> Gain/1  "va"
  Gain/1 -> Data Store Write3/1

== system npc_controller/CONTROL/GET_ADC/ADC/codegen/Subsystem2 ==
  adc : Inport
  Data Store Write3 : DataStoreWrite  DataStoreName=rms_vc  IndexOptions=Index vector (dialog)  Indices=1  OutputSizes=1
  Gain : Gain  Gain=1.11  ParamDataTypeStr=single  OutDataTypeStr=single
  IIR Filter1 : Subsystem
  Less Than : RelationalOperator  Operator=>  OutDataTypeStr=boolean  RndMeth=Simplest  InputSameDT=off
  Less Than1 : RelationalOperator  Operator=<  OutDataTypeStr=boolean  RndMeth=Simplest  InputSameDT=off
  Offset7 : Constant  Value=0  OutDataTypeStr=single
  Offset8 : Constant  Value=0  OutDataTypeStr=single
  Product : Product  OutDataTypeStr=single
  Product1 : Product  OutDataTypeStr=single
  vabc7 : Sum  Inputs=|+-  AccumDataTypeStr=single  OutDataTypeStr=single
  adc_rect : Outport
  wires:
  Less Than1/1 -> Product1/2
  Offset7/1 -> Less Than/2
  Offset8/1 -> Less Than1/2
  Less Than/1 -> Product/2
  Product/1 -> vabc7/1
  Product1/1 -> vabc7/2
  adc/1 -> Product1/1, Less Than1/1, Product/1, Less Than/1
  IIR Filter1/1(y[n]) -> Gain/1  "va"
  Gain/1 -> Data Store Write3/1
  vabc7/1 -> IIR Filter1/1(x[n]), adc_rect/1

== system npc_controller/CONTROL/GET_ADC/ADC/codegen/Subsystem3 ==
  adc : Inport
  Data Store Write3 : DataStoreWrite  DataStoreName=rms_ia  IndexOptions=Index vector (dialog)  Indices=1  OutputSizes=1
  Gain : Gain  Gain=1.11  ParamDataTypeStr=single  OutDataTypeStr=single
  IIR Filter1 : Subsystem
  Less Than : RelationalOperator  Operator=>  OutDataTypeStr=boolean  RndMeth=Simplest  InputSameDT=off
  Less Than1 : RelationalOperator  Operator=<  OutDataTypeStr=boolean  RndMeth=Simplest  InputSameDT=off
  Offset7 : Constant  Value=0  OutDataTypeStr=single
  Offset8 : Constant  Value=0  OutDataTypeStr=single
  Product : Product  OutDataTypeStr=single
  Product1 : Product  OutDataTypeStr=single
  vabc7 : Sum  Inputs=|+-  AccumDataTypeStr=single  OutDataTypeStr=single
  adc_rect : Outport
  wires:
  vabc7/1 -> IIR Filter1/1(x[n]), adc_rect/1
  adc/1 -> Less Than/1, Product/1, Less Than1/1, Product1/1
  Product1/1 -> vabc7/2
  Product/1 -> vabc7/1
  Less Than/1 -> Product/2
  Offset8/1 -> Less Than1/2
  Offset7/1 -> Less Than/2
  Less Than1/1 -> Product1/2
  IIR Filter1/1(y[n]) -> Gain/1  "va"
  Gain/1 -> Data Store Write3/1

== system npc_controller/CONTROL/GET_ADC/ADC/codegen/Subsystem4 ==
  adc : Inport
  Data Store Write3 : DataStoreWrite  DataStoreName=rms_ib  IndexOptions=Index vector (dialog)  Indices=1  OutputSizes=1
  Gain : Gain  Gain=1.11  ParamDataTypeStr=single  OutDataTypeStr=single
  IIR Filter1 : Subsystem
  Less Than : RelationalOperator  Operator=>  OutDataTypeStr=boolean  RndMeth=Simplest  InputSameDT=off
  Less Than1 : RelationalOperator  Operator=<  OutDataTypeStr=boolean  RndMeth=Simplest  InputSameDT=off
  Offset7 : Constant  Value=0  OutDataTypeStr=single
  Offset8 : Constant  Value=0  OutDataTypeStr=single
  Product : Product  OutDataTypeStr=single
  Product1 : Product  OutDataTypeStr=single
  vabc7 : Sum  Inputs=|+-  AccumDataTypeStr=single  OutDataTypeStr=single
  adc_rect : Outport
  wires:
  Less Than1/1 -> Product1/2
  Offset7/1 -> Less Than/2
  Offset8/1 -> Less Than1/2
  Less Than/1 -> Product/2
  Product/1 -> vabc7/1
  Product1/1 -> vabc7/2
  adc/1 -> Product1/1, Less Than1/1, Product/1, Less Than/1
  vabc7/1 -> IIR Filter1/1(x[n]), adc_rect/1
  IIR Filter1/1(y[n]) -> Gain/1  "va"
  Gain/1 -> Data Store Write3/1

== system npc_controller/CONTROL/GET_ADC/ADC/codegen/Subsystem5 ==
  adc : Inport
  Data Store Write3 : DataStoreWrite  DataStoreName=rms_ic  IndexOptions=Index vector (dialog)  Indices=1  OutputSizes=1
  Gain : Gain  Gain=1.11  ParamDataTypeStr=single  OutDataTypeStr=single
  IIR Filter1 : Subsystem
  Less Than : RelationalOperator  Operator=>  OutDataTypeStr=boolean  RndMeth=Simplest  InputSameDT=off
  Less Than1 : RelationalOperator  Operator=<  OutDataTypeStr=boolean  RndMeth=Simplest  InputSameDT=off
  Offset7 : Constant  Value=0  OutDataTypeStr=single
  Offset8 : Constant  Value=0  OutDataTypeStr=single
  Product : Product  OutDataTypeStr=single
  Product1 : Product  OutDataTypeStr=single
  vabc7 : Sum  Inputs=|+-  AccumDataTypeStr=single  OutDataTypeStr=single
  adc_rect : Outport
  wires:
  vabc7/1 -> IIR Filter1/1(x[n]), adc_rect/1
  adc/1 -> Less Than/1, Product/1, Less Than1/1, Product1/1
  Product1/1 -> vabc7/2
  Product/1 -> vabc7/1
  Less Than/1 -> Product/2
  Offset8/1 -> Less Than1/2
  Offset7/1 -> Less Than/2
  Less Than1/1 -> Product1/2
  IIR Filter1/1(y[n]) -> Gain/1  "va"
  Gain/1 -> Data Store Write3/1

== system npc_controller/CONTROL/GET_ADC/ADC/codegen/Subsystem6 ==
  note: ave to rms
  adc : Inport
  Data Store Write3 : DataStoreWrite  DataStoreName=rms_iphasea  IndexOptions=Index vector (dialog)  Indices=1  OutputSizes=1
  Gain : Gain  Gain=1.11  ParamDataTypeStr=single  OutDataTypeStr=single
  IIR Filter1 : Subsystem
  Less Than : RelationalOperator  Operator=>  OutDataTypeStr=boolean  RndMeth=Simplest  InputSameDT=off
  Less Than1 : RelationalOperator  Operator=<  OutDataTypeStr=boolean  RndMeth=Simplest  InputSameDT=off
  Offset7 : Constant  Value=0  OutDataTypeStr=single
  Offset8 : Constant  Value=0  OutDataTypeStr=single
  Product : Product  OutDataTypeStr=single
  Product1 : Product  OutDataTypeStr=single
  vabc7 : Sum  Inputs=|+-  AccumDataTypeStr=single  OutDataTypeStr=single
  wires:
  Gain/1 -> Data Store Write3/1
  IIR Filter1/1(y[n]) -> Gain/1  "va"
  vabc7/1 -> IIR Filter1/1(x[n])
  adc/1 -> Less Than/1, Product/1, Less Than1/1, Product1/1
  Product1/1 -> vabc7/2
  Product/1 -> vabc7/1
  Less Than/1 -> Product/2
  Offset8/1 -> Less Than1/2
  Offset7/1 -> Less Than/2
  Less Than1/1 -> Product1/2

== system npc_controller/CONTROL/GET_ADC/ADC/codegen/Subsystem7 ==
  adc : Inport
  Data Store Write3 : DataStoreWrite  DataStoreName=rms_iphaseb  IndexOptions=Index vector (dialog)  Indices=1  OutputSizes=1
  Gain : Gain  Gain=1.11  ParamDataTypeStr=single  OutDataTypeStr=single
  IIR Filter1 : Subsystem
  Less Than : RelationalOperator  Operator=>  OutDataTypeStr=boolean  RndMeth=Simplest  InputSameDT=off
  Less Than1 : RelationalOperator  Operator=<  OutDataTypeStr=boolean  RndMeth=Simplest  InputSameDT=off
  Offset7 : Constant  Value=0  OutDataTypeStr=single
  Offset8 : Constant  Value=0  OutDataTypeStr=single
  Product : Product  OutDataTypeStr=single
  Product1 : Product  OutDataTypeStr=single
  vabc7 : Sum  Inputs=|+-  AccumDataTypeStr=single  OutDataTypeStr=single
  wires:
  Gain/1 -> Data Store Write3/1
  IIR Filter1/1(y[n]) -> Gain/1  "va"
  Less Than1/1 -> Product1/2
  Offset7/1 -> Less Than/2
  Offset8/1 -> Less Than1/2
  Less Than/1 -> Product/2
  Product/1 -> vabc7/1
  Product1/1 -> vabc7/2
  adc/1 -> Product1/1, Less Than1/1, Product/1, Less Than/1
  vabc7/1 -> IIR Filter1/1(x[n])

== system npc_controller/CONTROL/GET_ADC/ADC/codegen/Subsystem8 ==
  adc : Inport
  Data Store Write3 : DataStoreWrite  DataStoreName=rms_iphasec  IndexOptions=Index vector (dialog)  Indices=1  OutputSizes=1
  Gain : Gain  Gain=1.11  ParamDataTypeStr=single  OutDataTypeStr=single
  IIR Filter1 : Subsystem
  Less Than : RelationalOperator  Operator=>  OutDataTypeStr=boolean  RndMeth=Simplest  InputSameDT=off
  Less Than1 : RelationalOperator  Operator=<  OutDataTypeStr=boolean  RndMeth=Simplest  InputSameDT=off
  Offset7 : Constant  Value=0  OutDataTypeStr=single
  Offset8 : Constant  Value=0  OutDataTypeStr=single
  Product : Product  OutDataTypeStr=single
  Product1 : Product  OutDataTypeStr=single
  vabc7 : Sum  Inputs=|+-  AccumDataTypeStr=single  OutDataTypeStr=single
  wires:
  vabc7/1 -> IIR Filter1/1(x[n])
  Gain/1 -> Data Store Write3/1
  IIR Filter1/1(y[n]) -> Gain/1  "va"
  adc/1 -> Less Than/1, Product/1, Less Than1/1, Product1/1
  Product1/1 -> vabc7/2
  Product/1 -> vabc7/1
  Less Than/1 -> Product/2
  Offset8/1 -> Less Than1/2
  Offset7/1 -> Less Than/2
  Less Than1/1 -> Product1/2

== system npc_controller/CONTROL/GET_ADC/ADC/sim/IIR Filter1 ==
  note: 10 half cycles of 50Hz
      |
      | 1/(5*650)
  note: prev 0.98
  x[n] : Inport
  1 - Lambda : Gain  Gain=0.00015384  ParamDataTypeStr=single  OutDataTypeStr=single
  Delay : Delay  DelayLength=1
  Lambda : Gain  Gain=0.99984615  ParamDataTypeStr=single  OutDataTypeStr=single
  Sum : Sum  Inputs=|++  AccumDataTypeStr=single  OutDataTypeStr=single
  y[n] : Outport
  wires:
  Delay/1 -> Lambda/1
  Lambda/1 -> Sum/2
  Sum/1 -> y[n]/1, Delay/1
  1 - Lambda/1 -> Sum/1
  x[n]/1 -> 1 - Lambda/1

== system npc_controller/CONTROL/GET_ADC/ADC/sim/IIR Filter3 ==
  note: prev 0.98
  x[n] : Inport
  1 - Lambda : Gain  Gain=1 - 0.95  ParamDataTypeStr=single  OutDataTypeStr=single
  Delay : Delay  DelayLength=1
  Lambda : Gain  Gain=0.95  ParamDataTypeStr=single  OutDataTypeStr=single
  Sum : Sum  Inputs=|++  AccumDataTypeStr=single  OutDataTypeStr=single
  y[n] : Outport
  wires:
  x[n]/1 -> 1 - Lambda/1
  1 - Lambda/1 -> Sum/1
  Sum/1 -> Delay/1, y[n]/1
  Lambda/1 -> Sum/2
  Delay/1 -> Lambda/1

== system npc_controller/CONTROL/GET_ADC/ADC/sim/IIR Filter5 ==
  note: prev 0.98
  x[n] : Inport
  1 - Lambda : Gain  Gain=1 - 0.95  ParamDataTypeStr=single  OutDataTypeStr=single
  Delay : Delay  DelayLength=1
  Lambda : Gain  Gain=0.95  ParamDataTypeStr=single  OutDataTypeStr=single
  Sum : Sum  Inputs=|++  AccumDataTypeStr=single  OutDataTypeStr=single
  y[n] : Outport
  wires:
  Delay/1 -> Lambda/1
  Lambda/1 -> Sum/2
  Sum/1 -> y[n]/1, Delay/1
  1 - Lambda/1 -> Sum/1
  x[n]/1 -> 1 - Lambda/1

== system npc_controller/CONTROL/GET_ADC/ADC/sim/IIR Filter8 ==
  note: prev 0.98
  x[n] : Inport
  1 - Lambda : Gain  Gain=1 - 0.95  ParamDataTypeStr=single  OutDataTypeStr=single
  Delay : Delay  DelayLength=1
  Lambda : Gain  Gain=0.95  ParamDataTypeStr=single  OutDataTypeStr=single
  Sum : Sum  Inputs=|++  AccumDataTypeStr=single  OutDataTypeStr=single
  y[n] : Outport
  wires:
  Delay/1 -> Lambda/1
  Lambda/1 -> Sum/2
  Sum/1 -> y[n]/1, Delay/1
  1 - Lambda/1 -> Sum/1
  x[n]/1 -> 1 - Lambda/1

== system npc_controller/CONTROL/GET_ADC/ADC/sim/Subsystem ==
  adc : Inport
  Less Than : RelationalOperator  Operator=>  OutDataTypeStr=boolean  RndMeth=Simplest  InputSameDT=off
  Less Than1 : RelationalOperator  Operator=<  OutDataTypeStr=boolean  RndMeth=Simplest  InputSameDT=off
  Offset7 : Constant  Value=0  OutDataTypeStr=single
  Offset8 : Constant  Value=0  OutDataTypeStr=single
  Product : Product  OutDataTypeStr=single
  Product1 : Product  OutDataTypeStr=single
  vabc7 : Sum  Inputs=|+-  AccumDataTypeStr=single  OutDataTypeStr=single
  adc_rect : Outport
  wires:
  Less Than1/1 -> Product1/2
  Offset7/1 -> Less Than/2
  Offset8/1 -> Less Than1/2
  Less Than/1 -> Product/2
  Product/1 -> vabc7/1
  Product1/1 -> vabc7/2
  adc/1 -> Product1/1, Less Than1/1, Product/1, Less Than/1
  vabc7/1 -> adc_rect/1

== system npc_controller/CONTROL/GET_ADC/ADC/sim/Subsystem1 ==
  adc : Inport
  Less Than : RelationalOperator  Operator=>  OutDataTypeStr=boolean  RndMeth=Simplest  InputSameDT=off
  Less Than1 : RelationalOperator  Operator=<  OutDataTypeStr=boolean  RndMeth=Simplest  InputSameDT=off
  Offset7 : Constant  Value=0  OutDataTypeStr=single
  Offset8 : Constant  Value=0  OutDataTypeStr=single
  Product : Product  OutDataTypeStr=single
  Product1 : Product  OutDataTypeStr=single
  vabc7 : Sum  Inputs=|+-  AccumDataTypeStr=single  OutDataTypeStr=single
  adc_rect : Outport
  wires:
  vabc7/1 -> adc_rect/1
  adc/1 -> Less Than/1, Product/1, Less Than1/1, Product1/1
  Product1/1 -> vabc7/2
  Product/1 -> vabc7/1
  Less Than/1 -> Product/2
  Offset8/1 -> Less Than1/2
  Offset7/1 -> Less Than/2
  Less Than1/1 -> Product1/2
